simulink model "ACCBase003_dist"  (Simulink 8.3)
settings: Solver=FixedStepDiscrete  StartTime=0.0  StopTime=10.0  FixedStep=0.1  RelTol=1e-3
model workspace (MAT data in the model file):
  pACC.Kp = 0.1
  pACC.minDist2Target = 50
  pACC.Ki = 0.0001
  pACC.KpDist = 1
  pACC.KiDist : numeric (value not decoded)
settings Model: Creator=swami  LastModifiedBy=swami
settings DataIOCC: SignalLoggingSaveFormat=Dataset
settings DebuggingCC: UnderspecifiedInitializationDetection=Simplified  StateNameClashWarn=none
settings GRTTargetCC: CombineOutputUpdateFcns=on  GRTInterface=off

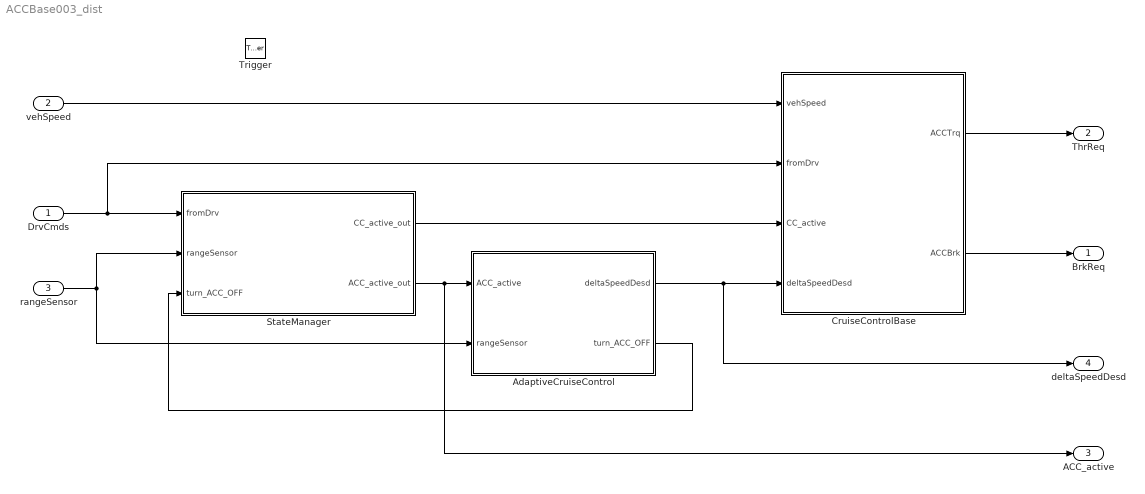
== system ACCBase003_dist ==
  DrvCmds : Inport  PortDimensions=4
  vehSpeed : Inport  Port=2
  rangeSensor : Inport  Port=3
  Trigger : TriggerPort  TriggerType=function-call  PortDimensions=1
  AdaptiveCruiseControl : MATLAB Function  TreatAsAtomicUnit=on
  CruiseControlBase : MATLAB Function  TreatAsAtomicUnit=on
  StateManager : MATLAB Function  TreatAsAtomicUnit=on
  BrkReq : Outport  PortDimensions=1
  ThrReq : Outport  Port=2  PortDimensions=1
  ACC_active : Outport  Port=3  PortDimensions=1
  deltaSpeedDesd : Outport  Port=4  PortDimensions=1
  wires:
  DrvCmds/1 -> StateManager/1(fromDrv), CruiseControlBase/2(fromDrv)
  rangeSensor/1 -> StateManager/2(rangeSensor), AdaptiveCruiseControl/2(rangeSensor)
  vehSpeed/1 -> CruiseControlBase/1(vehSpeed)
  StateManager/1(CC_active_out) -> CruiseControlBase/3(CC_active)
  CruiseControlBase/1(ACCTrq) -> ThrReq/1
  CruiseControlBase/2(ACCBrk) -> BrkReq/1
  StateManager/2(ACC_active_out) -> ACC_active/1, AdaptiveCruiseControl/1(ACC_active)
  AdaptiveCruiseControl/2(turn_ACC_OFF) -> StateManager/3(turn_ACC_OFF)
  AdaptiveCruiseControl/1(deltaSpeedDesd) -> deltaSpeedDesd/1, CruiseControlBase/4(deltaSpeedDesd)

== matlab function StateManager ==
  data: CC_active_out output double; fromDrv input double; ACC_active_out output double; rangeSensor input double; turn_ACC_OFF input double; pACC parameter double
function [CC_active_out,ACC_active_out] = fcn(fromDrv,rangeSensor,turn_ACC_OFF,pACC)
%#codegen
persistent dbgcnt;
persistent CC_active;
persistent ACC_active;
if isempty(ACC_active)
    CC_active = 0;
    ACC_active = 0;
    dbgcnt = 0;
end
dbgcnt = dbgcnt + 1;

DrvCCSw = fromDrv(3);

dist2Target = rangeSensor(1);

minDist2Target = pACC.minDist2Target;
ACCBuffer = minDist2Target * 0.9;
if DrvCCSw > 0.5
    if (CC_active == 0)
        CC_active = 1;
    end
    if (dist2Target < minDist2Target)
        % need to slow down
        ACC_active = 1;
    elseif (dist2Target > (minDist2Target + ACCBuffer))
        ACC_active = 0;
    end
    
    if (ACC_active == 1)            
        if turn_ACC_OFF > 0.5
            ACC_active = 0;
        end
    end
    
else
    CC_active = 0;
    ACC_active = 0;
end
ACC_active_out = ACC_active;
CC_active_out = CC_active;

== matlab function CruiseControlBase ==
  data: vehSpeed input double; fromDrv input double; CC_active input double; deltaSpeedDesd input double; ACCTrq output double; ACCBrk output double; pACC parameter double
function [ACCTrq,ACCBrk] = fcn(vehSpeed,fromDrv,CC_active,deltaSpeedDesd,pACC)
%#codegen
persistent torq_req_int;
persistent torq_req_old;
persistent CC_active_old;
if isempty(CC_active_old)    
    torq_req_int = 0;
    torq_req_old = 0;
end

DrvBrk = fromDrv(1);
DrvThr = fromDrv(2);
DrvCCSetPoint = fromDrv(4);

if CC_active > 0.5
        
   errorKp = (DrvCCSetPoint + deltaSpeedDesd - vehSpeed) * pACC.Kp;
   
   torq_req_int = torq_req_int + errorKp * pACC.Ki;    
   torq_req_prop = errorKp;   
   torq_req = torq_req_prop + torq_req_int;
   
   if (torq_req > 1.0)
       torq_req = 1.0;
   elseif (torq_req < -1.0)
       torq_req = -1.0;
   end    
   if torq_req < 0.0
       ACCBrk = 0.0 - torq_req;
       ACCTrq = 0.0;
   else
       ACCBrk = 0.0;
       ACCTrq = torq_req;
   end
else
    CC_active = 0;
    ACCTrq = DrvThr;
    ACCBrk = DrvBrk;
    torq_req = ACCTrq;
end
if ((CC_active_old ==0) && (CC_active == 1))
    torq_req_int = torq_req_old;
end

torq_req_old = torq_req;
CC_active_old = CC_active;

== matlab function AdaptiveCruiseControl ==
  data: ACC_active input double; rangeSensor input double; pACC parameter double; deltaSpeedDesd output double; turn_ACC_OFF output double
function [deltaSpeedDesd, turn_ACC_OFF]  = fcn(ACC_active,rangeSensor, pACC)
%#codegen
persistent ACC_active_old;
persistent errorKiDist;
if isempty(ACC_active_old)
    errorKiDist = 0;
end

dist2Target = rangeSensor(1);
minDist2Target = pACC.minDist2Target;
turn_ACC_OFF = 0;

if (ACC_active == 1)
    errorKpDist = (dist2Target - minDist2Target) * pACC.KpDist;
    errorKiDist = errorKiDist + errorKpDist * pACC.KiDist;
    deltaSpeedDesd = errorKpDist + errorKiDist;
    
    if deltaSpeedDesd > 0.0
        deltaSpeedDesd = 0;
        turn_ACC_OFF = 1;
    end

else
    deltaSpeedDesd = 0;
end
    
if ((ACC_active_old ==0) && (ACC_active == 1))
    errorKiDist = 0;
end
ACC_active_old = ACC_active;
